simulink model "p4_car_colton_update1"  (R2025a)
settings: Solver=ode5  StartTime=0.0  StopTime=3600  FixedStep=0.001  RelTol=1e-3
undefined symbols (not defined in the file or in its folder): datBat, datCar, datMotor, path
libraries: slpidlib x1
settings Model: Creator=dxego  LastModifiedBy=umar
settings OptimizationCC: ReuseModelBlockBuffer=off
settings RTWCC: GPUComputeCapability=3.5

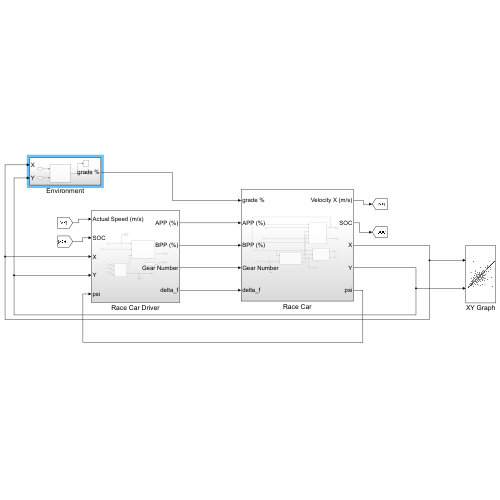
[thumbnail: Simulink's stored preview of the top-level diagram]
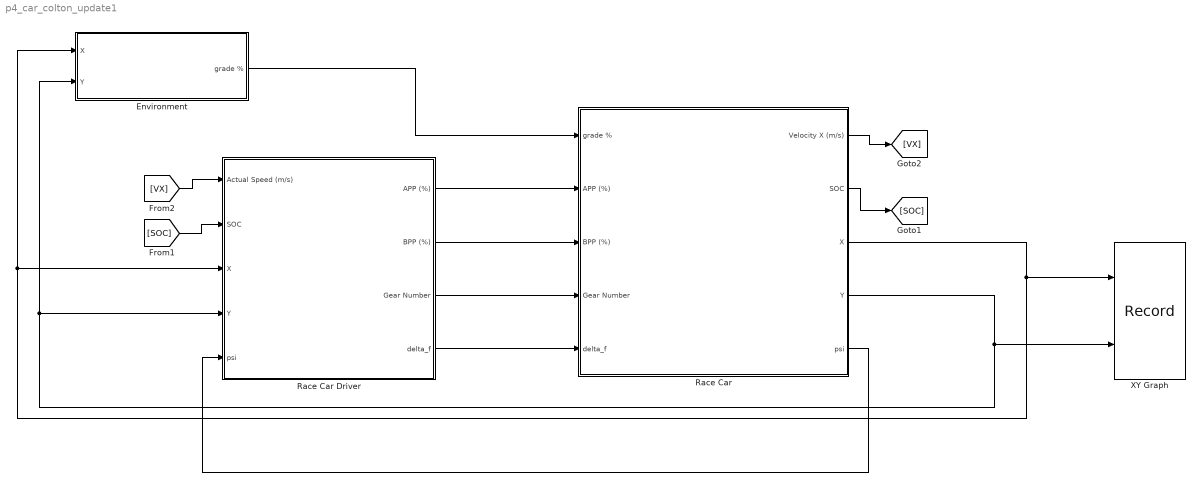
== system p4_car_colton_update1 ==
  Environment : Subsystem
  Race Car : Subsystem
  Race Car Driver : Subsystem
  XY Graph : Record  NumPorts=2.0  FileSettingsInternal="{\"entries\":[{\"content\":{\"excelSettings\":{\"content\":{},\"type\":\"Streamout.ExcelSettings\"},\"parquetSettings\":{\"content\":{},\"type\":\"Streamout.ParquetSettings\"}},\"type\":\"Streamout.FileSettingStorage\",\"uuid\":\"\"}],\"packageUris\":[\"http:\\/\\/schema.mathworks.com\\/mf0\\/streamout_blocks\\/R2020a\"],\"version\":\"1.0\"}"  FrameSettings=[0, 0]  Layout=[1 1]  SignalsInternal="{\"entries\":[{\"content\":{\"signals\":[{\"content\":{\"blockPath\":[],\"dimensions\":[1],\"domain\":\"\",\"lineColor\":\"#a2142f\",\"plots\":[ 1 ],\"port\":1,\"sid\":[\"\"],\"signalID\":1,\"signalName\":\"Race Car:3\"},\"type\":\"RecordBlkView.Signal\",\"uuid\":\"\"},{\"content\":{\"blockPath\":[],\"dimensions\":[1],\"domain\":\"\",\"lineColor\":\"#139fff\",\"plots\":[ 1 ],\"port\":2,\"sid\":[\"\"],\"signalID\":2,\"signalName\":\"Race Car:4\"},\"type\":\"RecordBlkView.Signal\",\"uuid\":\"\"}]},\"type\":\"RecordBlkView.InputSignals\",\"uuid\":\"\"}],\"packageUris\":[\"http:\\/\\/schema.mathworks.com\\/mf0\\/streamout_blocks\\/R2020a\"],\"version\":\"1.0\"}"  VisualizationBindings="{\"xyplotplugin\":{\"info\":[{\"series\":[{\"bindingParametersList\":[{\"parameter\":\"X-Axis\",\"signalID\":1,\"signalName\":\"Race Car:3\"},{\"parameter\":\"Y-Axis\",\"signalID\":2,\"signalName\":\"Race Car:4\"}],\"seriesID\":0}],\"subplotID\":1}]}}"  CompatibilityTag=XY  st=-1
  wires:
  [VX] -> Race Car Driver/1(Actual Speed (m/s))
  [SOC] -> Race Car Driver/2(SOC)
  Race Car/4(Y) -> XY Graph/2, Environment/2(Y), Race Car Driver/4(Y)
  Race Car/3(X) -> XY Graph/1, Environment/1(X), Race Car Driver/3(X)
  Race Car Driver/1(APP (%)) -> Race Car/2(APP (%))
  Race Car Driver/2(BPP (%)) -> Race Car/3("BPP (%) ")
  Race Car Driver/4(delta_f) -> Race Car/5(delta_f)
  Race Car/1(Velocity X (m/s)) -> [VX]
  Race Car/2(SOC) -> [SOC]
  Race Car Driver/3(Gear Number) -> Race Car/4(Gear Number)
  Environment/1(grade %) -> Race Car/1(grade %)
  Race Car/5(psi) -> Race Car Driver/5(psi)

== system p4_car_colton_update1/Environment ==
  X : Inport
  Y : Inport  Port=2
  MATLAB Function : MATLAB Function  TreatAsAtomicUnit=on
  Scope : Scope
      settings: ActiveDisplayYMinimum=-0.037768533551662917  ActiveDisplayYMaximum=0.038970623034102633  DataLoggingVariableName=ScopeData19
  grade % : Outport
  wires:
  X/1 -> MATLAB Function/1(x)
  Y/1 -> MATLAB Function/2(y)
  MATLAB Function/1(g) -> Scope/1, grade %/1

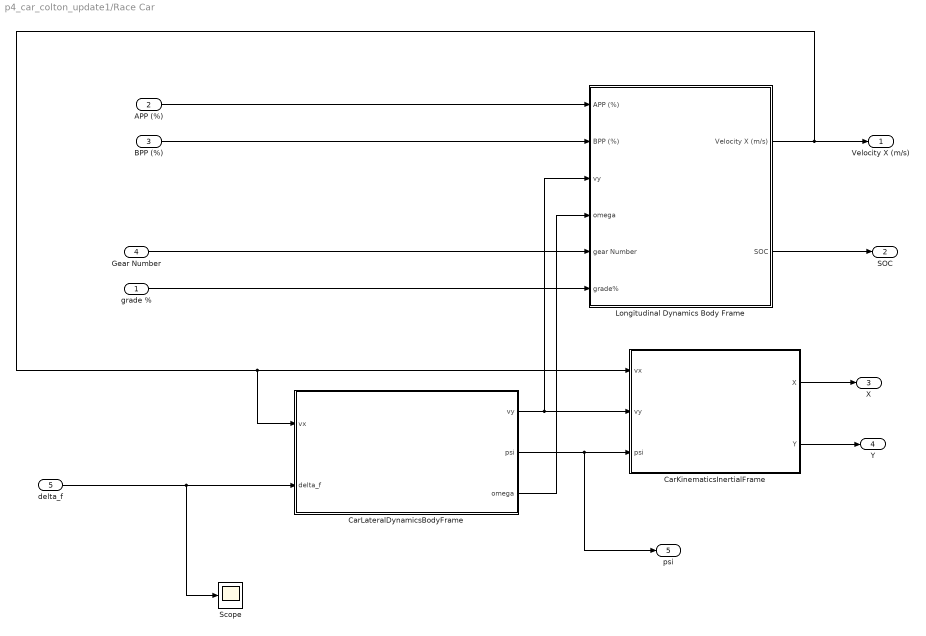
== system p4_car_colton_update1/Race Car ==
  grade % : Inport
  APP (%) : Inport  Port=2
  "BPP (%) " : Inport  Port=3
  Gear Number : Inport  Port=4
  delta_f : Inport  Port=5
  CarKinematicsInertialFrame : Subsystem
  CarLateralDynamicsBodyFrame : Subsystem
  Longitudinal Dynamics Body Frame : Subsystem
  Scope : Scope
      settings: ActiveDisplayYMinimum=-1.3496608820575011  ActiveDisplayYMaximum=9.010651011668978  DataLoggingVariableName=ScopeData16
  Velocity X (m/s) : Outport
  SOC : Outport  Port=2
  X : Outport  Port=3
  Y : Outport  Port=4
  psi : Outport  Port=5
  wires:
  CarKinematicsInertialFrame/2(Y) -> Y/1
  Longitudinal Dynamics Body Frame/2(SOC) -> SOC/1
  CarLateralDynamicsBodyFrame/2(psi) -> psi/1, CarKinematicsInertialFrame/3(psi)
  delta_f/1 -> Scope/1, CarLateralDynamicsBodyFrame/2(delta_f)
  APP (%)/1 -> Longitudinal Dynamics Body Frame/1(APP (%))
  CarLateralDynamicsBodyFrame/1(vy) -> Longitudinal Dynamics Body Frame/3(vy), CarKinematicsInertialFrame/2(vy)
  CarLateralDynamicsBodyFrame/3(omega) -> Longitudinal Dynamics Body Frame/4(omega)
  "BPP (%) "/1 -> Longitudinal Dynamics Body Frame/2("BPP (%) ")
  Longitudinal Dynamics Body Frame/1(Velocity X (m/s)) -> Velocity X (m/s)/1, CarLateralDynamicsBodyFrame/1(vx), CarKinematicsInertialFrame/1(vx)
  CarKinematicsInertialFrame/1(X) -> X/1
  Gear Number/1 -> Longitudinal Dynamics Body Frame/5(gear Number)
  grade %/1 -> Longitudinal Dynamics Body Frame/6(grade%)

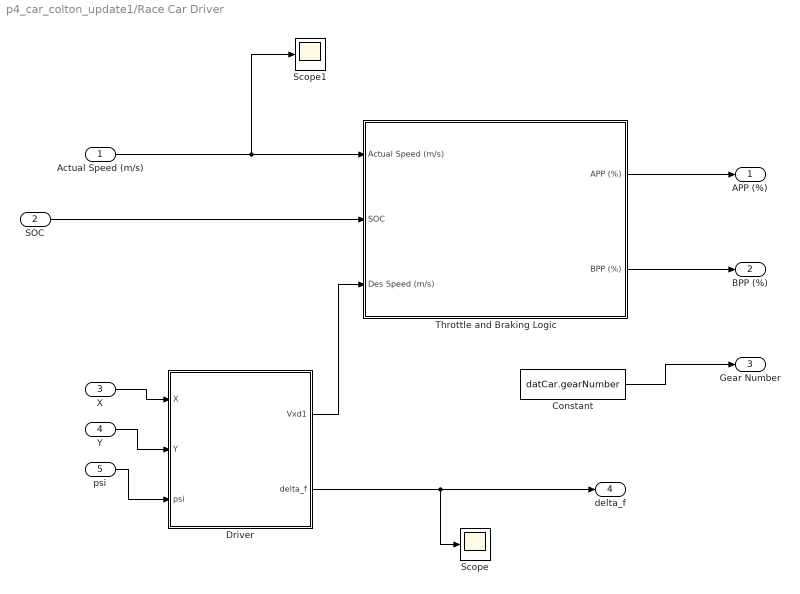
== system p4_car_colton_update1/Race Car Driver ==
  Actual Speed (m/s) : Inport
  SOC : Inport  Port=2
  X : Inport  Port=3
  Y : Inport  Port=4
  psi : Inport  Port=5
  Constant : Constant  Value=datCar.gearNumber
  Driver : Subsystem
  Scope : Scope
      settings: ActiveDisplayYMinimum=-1  ActiveDisplayYMaximum=1  DataLoggingVariableName=ScopeData12
  Scope1 : Scope
      settings: ActiveDisplayYMinimum=11.033893227651333  ActiveDisplayYMaximum=28.405080062704929  DataLoggingVariableName=ScopeData14
  "Throttle and Braking Logic " : Subsystem
  APP (%) : Outport
  BPP (%) : Outport  Port=2
  Gear Number : Outport  Port=3
  delta_f : Outport  Port=4
  wires:
  Y/1 -> Driver/2(Y)
  X/1 -> Driver/1(X)
  "Throttle and Braking Logic "/2(BPP (%)) -> BPP (%)/1
  Actual Speed (m/s)/1 -> Scope1/1, "Throttle and Braking Logic "/1(Actual Speed (m/s))
  "Throttle and Braking Logic "/1(APP (%)) -> APP (%)/1
  SOC/1 -> "Throttle and Braking Logic "/2(SOC)
  Driver/1(Vxd1) -> "Throttle and Braking Logic "/3("Des Speed (m/s) ")
  psi/1 -> Driver/3(psi)
  Constant/1 -> Gear Number/1
  Driver/2(delta_f) -> Scope/1, delta_f/1

== system p4_car_colton_update1/Race Car/CarKinematicsInertialFrame ==
  vx : Inport
  vy : Inport  Port=2
  psi : Inport  Port=3
  Integrator : Integrator  InitialCondition=datCar.init.X0
  Integrator1 : Integrator  InitialCondition=datCar.init.Y0
  KinematicVehicleModel_derivatives : MATLAB Function  TreatAsAtomicUnit=on  mask{obj=datCar}
      mask prompts: obj "obj structure"
  To Workspace : ToWorkspace  VariableName=X  SaveFormat=Timeseries  SampleTime=-1
  To Workspace1 : ToWorkspace  VariableName=Y  SaveFormat=Timeseries  SampleTime=-1
  X : Outport
  Y : Outport  Port=2
  wires:
  KinematicVehicleModel_derivatives/1(Xdot) -> Integrator/1
  KinematicVehicleModel_derivatives/2(Ydot) -> Integrator1/1
  Integrator/1 -> To Workspace/1, X/1
  Integrator1/1 -> Y/1, To Workspace1/1
  vx/1 -> KinematicVehicleModel_derivatives/1(vx)
  vy/1 -> KinematicVehicleModel_derivatives/2(vy)
  psi/1 -> KinematicVehicleModel_derivatives/3(psi)

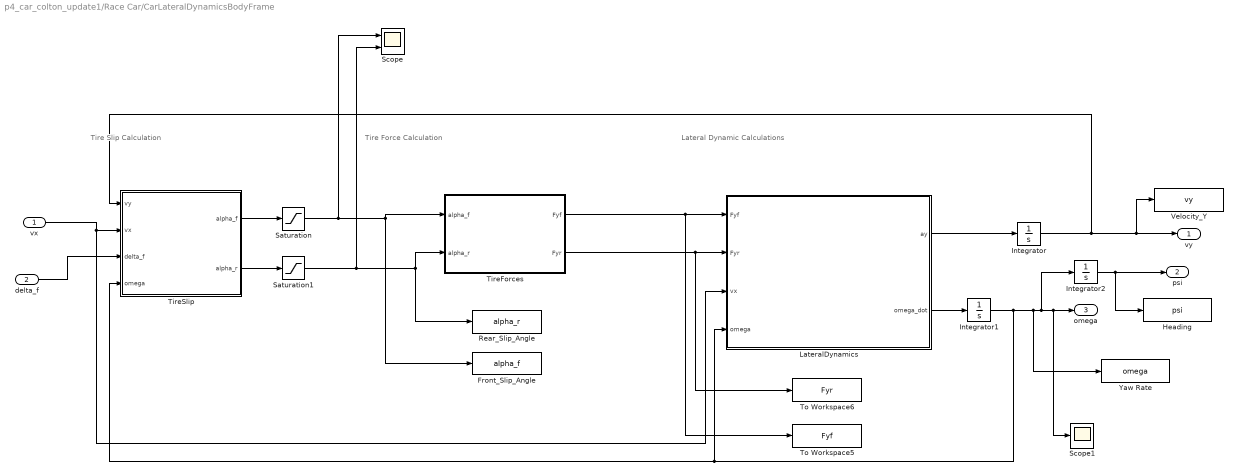
== system p4_car_colton_update1/Race Car/CarLateralDynamicsBodyFrame ==
  note: Tire Slip Calculation
  note: Tire Force Calculation
  note: Lateral Dynamic Calculations
  vx : Inport
  delta_f : Inport  Port=2
  Front_Slip_Angle : ToWorkspace  VariableName=alpha_f  SaveFormat=Timeseries  SampleTime=-1
  Heading : ToWorkspace  VariableName=psi  SaveFormat=Timeseries  SampleTime=-1
  Integrator : Integrator  InitialCondition=datCar.init.vy0
  Integrator1 : Integrator  InitialCondition=datCar.init.omega0
  Integrator2 : Integrator  InitialCondition=datCar.init.psi0
  LateralDynamics : MATLAB Function  TreatAsAtomicUnit=on  mask{obj=datCar}
      mask prompts: obj "obj structure"
  Rear_Slip_Angle : ToWorkspace  VariableName=alpha_r  SaveFormat=Timeseries  SampleTime=-1
  Saturation : Saturate  UpperLimit=datCar.maxAlpha  LowerLimit=-datCar.maxAlpha
  Saturation1 : Saturate  UpperLimit=datCar.maxAlpha  LowerLimit=-datCar.maxAlpha
  Scope : Scope  NumInputPorts=2
      settings: ActiveDisplayYMinimum=-1  ActiveDisplayYMaximum=1  DataLoggingVariableName=ScopeData13
  Scope1 : Scope
      settings: ActiveDisplayYMinimum=-1  ActiveDisplayYMaximum=1  DataLoggingVariableName=ScopeData17
  TireForces : MATLAB Function  TreatAsAtomicUnit=on  mask{obj=datCar}
      mask prompts: obj "obj structure"
  TireSlip : MATLAB Function  TreatAsAtomicUnit=on  mask{obj=datCar}
      mask prompts: obj "obj structure"
  To Workspace5 : ToWorkspace  VariableName=Fyf  SaveFormat=Timeseries  SampleTime=-1
  To Workspace6 : ToWorkspace  VariableName=Fyr  SaveFormat=Timeseries  SampleTime=-1
  Velocity_Y : ToWorkspace  VariableName=vy  SaveFormat=Timeseries  SampleTime=-1
  Yaw Rate : ToWorkspace  VariableName=omega  SaveFormat=Timeseries  SampleTime=-1
  vy : Outport
  psi : Outport  Port=2
  omega : Outport  Port=3
  wires:
  LateralDynamics/1(ay) -> Integrator/1
  Integrator/1 -> vy/1, Velocity_Y/1, TireSlip/1(vy)
  LateralDynamics/2(omega_dot) -> Integrator1/1
  Integrator1/1 -> Integrator2/1, Scope1/1, omega/1, Yaw Rate/1, LateralDynamics/4(omega), TireSlip/4(omega)
  TireSlip/1(alpha_f) -> Saturation/1
  TireSlip/2(alpha_r) -> Saturation1/1
  TireForces/1(Fyf) -> LateralDynamics/1(Fyf), To Workspace5/1
  TireForces/2(Fyr) -> LateralDynamics/2(Fyr), To Workspace6/1
  Saturation/1 -> Scope/1, TireForces/1(alpha_f), Front_Slip_Angle/1
  Saturation1/1 -> Scope/2, TireForces/2(alpha_r), Rear_Slip_Angle/1
  vx/1 -> TireSlip/2(vx), LateralDynamics/3(vx)
  delta_f/1 -> TireSlip/3(delta_f)
  Integrator2/1 -> Heading/1, psi/1

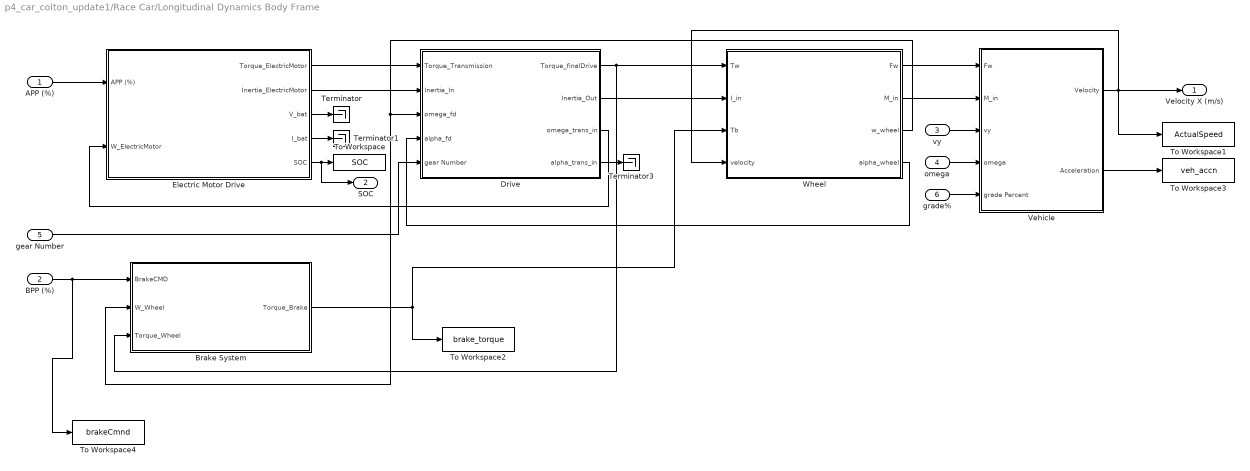
== system p4_car_colton_update1/Race Car/Longitudinal Dynamics Body Frame ==
  APP (%) : Inport
  "BPP (%) " : Inport  Port=2
  vy : Inport  Port=3
  omega : Inport  Port=4
  gear Number : Inport  Port=5
  grade% : Inport  Port=6
  Brake System : Subsystem
  Drive : Subsystem
  Electric Motor Drive : Subsystem
  Terminator : Terminator
  Terminator1 : Terminator
  Terminator3 : Terminator
  To Workspace : ToWorkspace  VariableName=SOC  SaveFormat=Timeseries  SampleTime=-1
  To Workspace1 : ToWorkspace  VariableName=ActualSpeed  SaveFormat=Timeseries  SampleTime=-1
  To Workspace2 : ToWorkspace  VariableName=brake_torque  SaveFormat=Timeseries  SampleTime=-1
  To Workspace3 : ToWorkspace  VariableName=veh_accn  SaveFormat=Timeseries  SampleTime=-1
  To Workspace4 : ToWorkspace  VariableName=brakeCmnd  SaveFormat=Timeseries  SampleTime=-1
  Vehicle : Subsystem
  "Wheel " : Subsystem
  Velocity X (m/s) : Outport
  SOC : Outport  Port=2
  wires:
  Drive/3(omega_trans_in) -> Electric Motor Drive/2(W_ElectricMotor)
  Electric Motor Drive/2(Inertia_ElectricMotor) -> Drive/2(Inertia_In)
  Electric Motor Drive/3(V_bat) -> Terminator/1
  Vehicle/2(Acceleration) -> To Workspace3/1
  Drive/1(Torque_finalDrive) -> "Wheel "/1(Tw), Brake System/3(Torque_Wheel)
  Electric Motor Drive/1(Torque_ElectricMotor) -> Drive/1(Torque_Transmission)
  Drive/2(Inertia_Out) -> "Wheel "/2(I_in)
  "Wheel "/2(M_in) -> Vehicle/2("M_in ")
  "BPP (%) "/1 -> To Workspace4/1, Brake System/1("BrakeCMD ")
  "Wheel "/3(w_wheel) -> Brake System/2(W_Wheel), Drive/3(omega_fd)
  "Wheel "/1(Fw) -> Vehicle/1(Fw)
  Brake System/1(Torque_Brake) -> To Workspace2/1, "Wheel "/3(Tb)
  Drive/4(alpha_trans_in) -> Terminator3/1
  "Wheel "/4(alpha_wheel) -> Drive/4(alpha_fd)
  Electric Motor Drive/4(I_bat) -> Terminator1/1
  APP (%)/1 -> Electric Motor Drive/1(APP (%))
  vy/1 -> Vehicle/3(vy)
  omega/1 -> Vehicle/4(omega)
  Vehicle/1("Velocity ") -> "Wheel "/4(velocity), Velocity X (m/s)/1, To Workspace1/1
  Electric Motor Drive/5(SOC) -> SOC/1, To Workspace/1
  gear Number/1 -> Drive/5(gear Number)
  grade%/1 -> Vehicle/5(grade Percent)

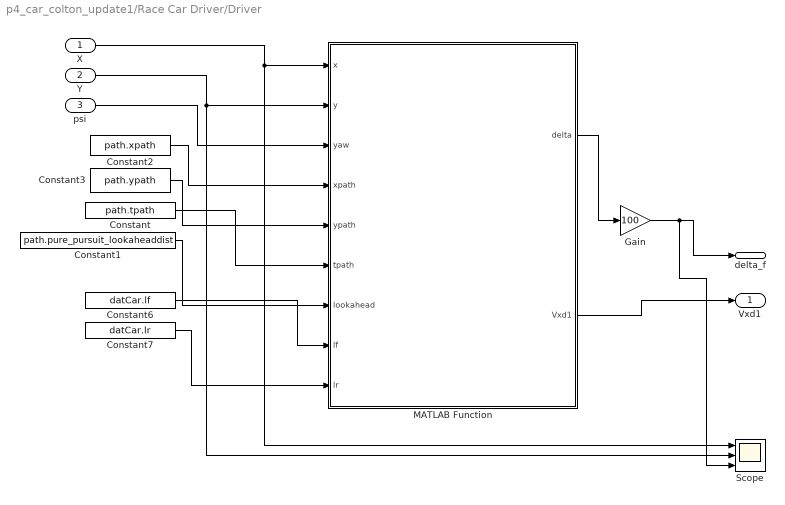
== system p4_car_colton_update1/Race Car Driver/Driver ==
  X : Inport
  Y : Inport  Port=2
  psi : Inport  Port=3
  Constant : Constant  Value=path.tpath
  Constant1 : Constant  Value=path.pure_pursuit_lookaheaddist
  Constant2 : Constant  Value=path.xpath
  Constant3 : Constant  Value=path.ypath
  Constant6 : Constant  Value=datCar.lf
  Constant7 : Constant  Value=datCar.lr
  Gain : Gain  Gain=100
  MATLAB Function : MATLAB Function  TreatAsAtomicUnit=on
  Scope : Scope  NumInputPorts=3
      settings: ActiveDisplayYMinimum=-137.49213624230239  ActiveDisplayYMaximum=1237.4292261807218
  Vxd1 : Outport
  delta_f : Outport  Port=2
  wires:
  X/1 -> Scope/1, MATLAB Function/1(x)
  Y/1 -> Scope/2, MATLAB Function/2(y)
  psi/1 -> MATLAB Function/3(yaw)
  MATLAB Function/2(Vxd1) -> Vxd1/1
  Constant2/1 -> MATLAB Function/4(xpath)
  Constant3/1 -> MATLAB Function/5(ypath)
  Constant/1 -> MATLAB Function/6(tpath)
  Constant1/1 -> MATLAB Function/7(lookahead)
  Constant6/1 -> MATLAB Function/8(lf)
  Constant7/1 -> MATLAB Function/9(lr)
  MATLAB Function/1(delta) -> Gain/1
  Gain/1 -> Scope/3, delta_f/1

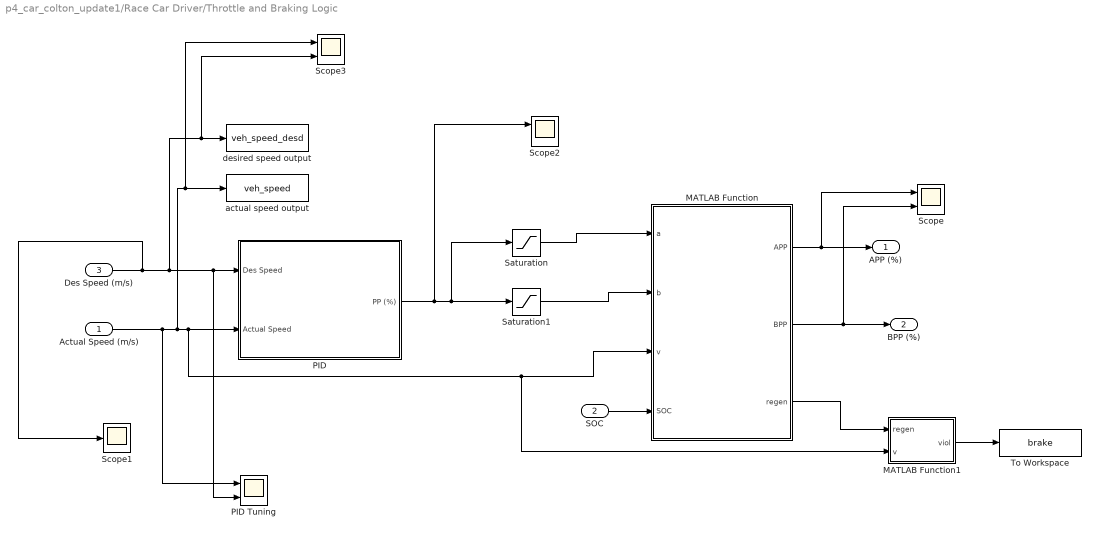
== system p4_car_colton_update1/Race Car Driver/Throttle and Braking Logic  ==
  Actual Speed (m/s) : Inport
  SOC : Inport  Port=2
  "Des Speed (m/s) " : Inport  Port=3
  MATLAB Function : MATLAB Function  TreatAsAtomicUnit=on
  MATLAB Function1 : MATLAB Function  TreatAsAtomicUnit=on
  PID : Subsystem
  PID Tuning : Scope  NumInputPorts=2
      settings: ActiveDisplayYMinimum=-4.40832  ActiveDisplayYMaximum=37.63006
  Saturation : Saturate  UpperLimit=1  LowerLimit=0
  Saturation1 : Saturate  UpperLimit=0  LowerLimit=-1
  Scope : Scope  NumInputPorts=2
      settings: ActiveDisplayYMinimum=-1.0607  ActiveDisplayYMaximum=1.06103
  Scope1 : Scope
      settings: ActiveDisplayYMinimum=-1  ActiveDisplayYMaximum=1  DataLoggingVariableName=ScopeData15
  Scope2 : Scope  NumInputPorts=2
      settings: ActiveDisplayYMinimum=-1.0607  ActiveDisplayYMaximum=1.06103  DataLoggingVariableName=ScopeData5
  Scope3 : Scope  NumInputPorts=2
      settings: ActiveDisplayYMinimum=27.321282013339456  ActiveDisplayYMaximum=39.0725745132226  DataLoggingVariableName=ScopeData11
  To Workspace : ToWorkspace  VariableName=brake  SaveFormat=Timeseries  SampleTime=-1
  actual speed output : ToWorkspace  VariableName=veh_speed  SaveFormat=Timeseries  SampleTime=-1
  desired speed output : ToWorkspace  VariableName=veh_speed_desd  SaveFormat=Timeseries  SampleTime=-1
  APP (%) : Outport
  BPP (%) : Outport  Port=2
  wires:
  PID/1(PP (%)) -> Scope2/1, Saturation1/1, Saturation/1
  Saturation1/1 -> MATLAB Function/2(b)
  Actual Speed (m/s)/1 -> PID Tuning/1, actual speed output/1, Scope3/1, MATLAB Function1/2(v), MATLAB Function/3(v), PID/2(Actual Speed)
  "Des Speed (m/s) "/1 -> Scope1/1, PID Tuning/2, PID/1("Des Speed "), Scope3/2, desired speed output/1
  Saturation/1 -> MATLAB Function/1(a)
  MATLAB Function/1(APP) -> Scope/1, APP (%)/1
  MATLAB Function/2(BPP) -> Scope/2, BPP (%)/1
  MATLAB Function1/1(viol) -> To Workspace/1
  SOC/1 -> MATLAB Function/4(SOC)
  MATLAB Function/3(regen) -> MATLAB Function1/1(regen)

== system p4_car_colton_update1/Race Car/Longitudinal Dynamics Body Frame/Brake System ==
  "BrakeCMD " : Inport
  W_Wheel : Inport  Port=2
  Torque_Wheel : Inport  Port=3
  Brake Torque : MATLAB Function  TreatAsAtomicUnit=on
  Constant : Constant  Value=datCar.maxBrakeTorque
  Scope : Scope
      settings: ActiveDisplayYMinimum=-3252.17168  ActiveDisplayYMaximum=56.62718  DataLoggingVariableName=ScopeData4
  Torque_Brake : Outport  VectorParamsAs1DForOutWhenUnconnected=off
  wires:
  "BrakeCMD "/1 -> Brake Torque/1(BBcmd)
  Brake Torque/1(Tb) -> Scope/1, Torque_Brake/1
  W_Wheel/1 -> Brake Torque/3(w_wheel)
  Constant/1 -> Brake Torque/2(Tbcap)

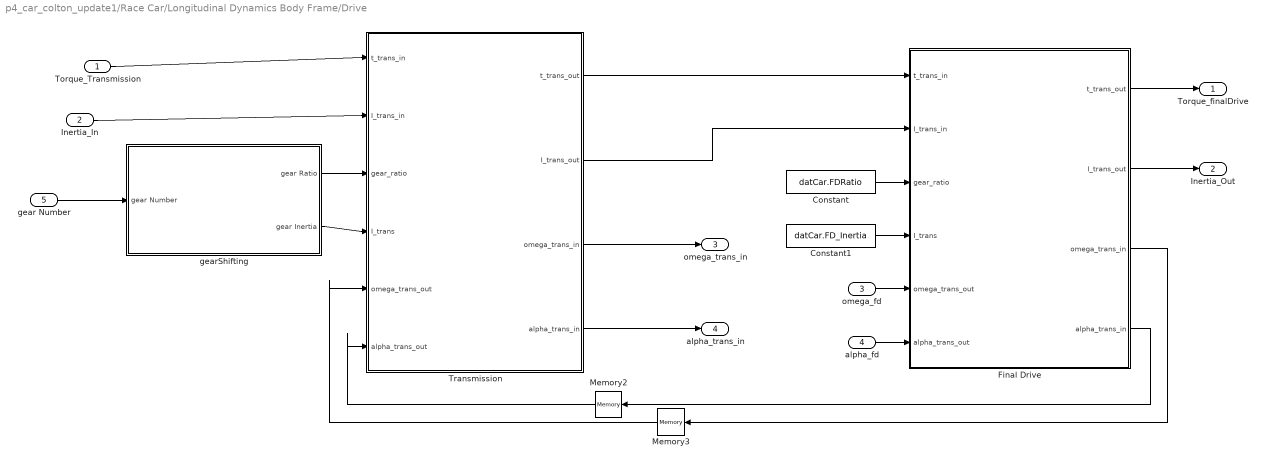
== system p4_car_colton_update1/Race Car/Longitudinal Dynamics Body Frame/Drive ==
  Torque_Transmission : Inport
  Inertia_In : Inport  Port=2
  omega_fd : Inport  Port=3
  alpha_fd : Inport  Port=4
  gear Number : Inport  Port=5
  Constant : Constant  Value=datCar.FDRatio
  Constant1 : Constant  Value=datCar.FD_Inertia
  Final Drive : MATLAB Function  TreatAsAtomicUnit=on
  Memory2 : Memory
  Memory3 : Memory
  Transmission : MATLAB Function  TreatAsAtomicUnit=on
  gearShifting : Subsystem
  Torque_finalDrive : Outport
  Inertia_Out : Outport  Port=2
  omega_trans_in : Outport  Port=3
  alpha_trans_in : Outport  Port=4
  wires:
  Final Drive/4(alpha_trans_in) -> Memory2/1
  Final Drive/3(omega_trans_in) -> Memory3/1
  Transmission/1(t_trans_out) -> Final Drive/1(t_trans_in)
  Transmission/2(I_trans_out) -> Final Drive/2(I_trans_in)
  Transmission/4(alpha_trans_in) -> alpha_trans_in/1
  Final Drive/1(t_trans_out) -> Torque_finalDrive/1
  Final Drive/2(I_trans_out) -> Inertia_Out/1
  omega_fd/1 -> Final Drive/5(omega_trans_out)
  alpha_fd/1 -> Final Drive/6(alpha_trans_out)
  Constant/1 -> Final Drive/3(gear_ratio)
  Constant1/1 -> Final Drive/4(I_trans)
  gear Number/1 -> gearShifting/1(gear Number)
  gearShifting/1(gear Ratio) -> Transmission/3(gear_ratio)
  gearShifting/2(gear Inertia) -> Transmission/4(I_trans)
  Inertia_In/1 -> Transmission/2(I_trans_in)
  Transmission/3(omega_trans_in) -> omega_trans_in/1
  Torque_Transmission/1 -> Transmission/1(t_trans_in)
  Memory2/1 -> Transmission/6(alpha_trans_out)
  Memory3/1 -> Transmission/5(omega_trans_out)

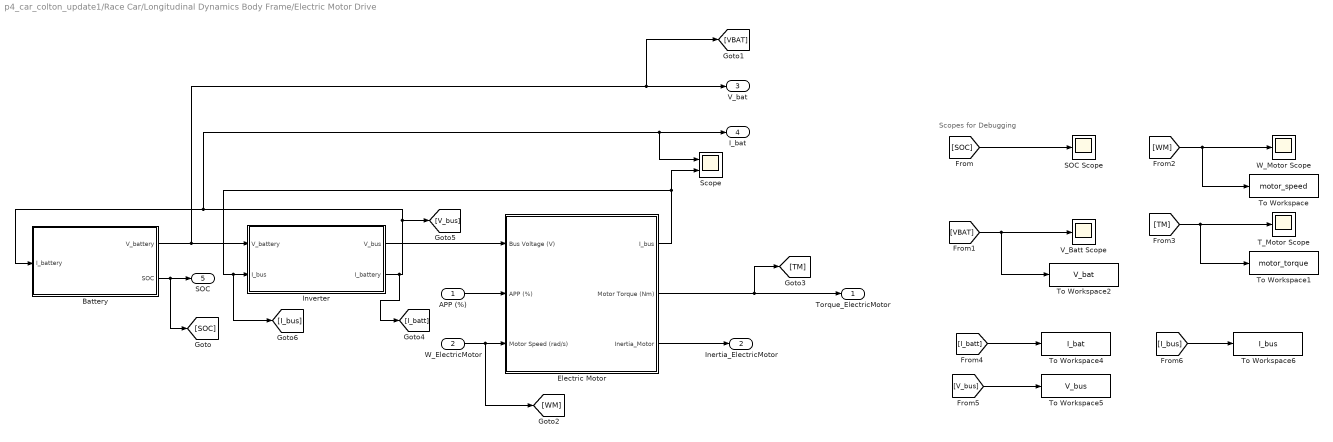
== system p4_car_colton_update1/Race Car/Longitudinal Dynamics Body Frame/Electric Motor Drive ==
  note: Scopes for Debugging
  APP (%) : Inport
  W_ElectricMotor : Inport  Port=2
  Battery : Subsystem
  Electric Motor : Subsystem
  Inverter : Subsystem
  SOC Scope : Scope
      settings: ActiveDisplayYMinimum=0.79068  ActiveDisplayYMaximum=0.80103  DataLoggingVariableName=ScopeData7
  Scope : Scope  NumInputPorts=2
      settings: ActiveDisplayYMinimum=-92.41521  ActiveDisplayYMaximum=118.26537  DataLoggingVariableName=ScopeData2
  T_Motor Scope : Scope
      settings: ActiveDisplayYMinimum=-92.74121  ActiveDisplayYMaximum=115.47111  DataLoggingVariableName=ScopeData10
  To Workspace : ToWorkspace  VariableName=motor_speed  SaveFormat=Timeseries  SampleTime=-1
  To Workspace1 : ToWorkspace  VariableName=motor_torque  SaveFormat=Timeseries  SampleTime=-1
  To Workspace2 : ToWorkspace  VariableName=V_bat  SaveFormat=Timeseries  SampleTime=-1
  To Workspace4 : ToWorkspace  VariableName=I_bat  SaveFormat=Timeseries  SampleTime=-1
  To Workspace5 : ToWorkspace  VariableName=V_bus  SaveFormat=Timeseries  SampleTime=-1
  To Workspace6 : ToWorkspace  VariableName=I_bus  SaveFormat=Timeseries  SampleTime=-1
  V_Batt Scope : Scope
      settings: ActiveDisplayYMinimum=354.15627  ActiveDisplayYMaximum=391.49042  DataLoggingVariableName=ScopeData8
  W_Motor Scope : Scope
      settings: ActiveDisplayYMinimum=-83.74997  ActiveDisplayYMaximum=695.87961  DataLoggingVariableName=ScopeData9
  Torque_ElectricMotor : Outport
  Inertia_ElectricMotor : Outport  Port=2
  V_bat : Outport  Port=3
  I_bat : Outport  Port=4
  SOC : Outport  Port=5
  wires:
  APP (%)/1 -> Electric Motor/2(APP (%))
  W_ElectricMotor/1 -> [WM], Electric Motor/3(Motor Speed (rad/s))
  Electric Motor/3(Inertia_Motor) -> Inertia_ElectricMotor/1
  Inverter/1(V_bus) -> Electric Motor/1(Bus Voltage (V))
  Inverter/2(I_battery) -> [I_batt], Scope/1, I_bat/1, Battery/1(I_battery), [V_bus]
  Electric Motor/1(I_bus) -> Scope/2, [I_bus], Inverter/2(I_bus)
  [SOC] -> SOC Scope/1
  [VBAT] -> To Workspace2/1, V_Batt Scope/1
  [WM] -> To Workspace/1, W_Motor Scope/1
  [TM] -> To Workspace1/1, T_Motor Scope/1
  Battery/1(V_battery) -> [VBAT], V_bat/1, Inverter/1(V_battery)
  Electric Motor/2(Motor Torque (Nm)) -> [TM], Torque_ElectricMotor/1
  Battery/2(SOC) -> [SOC], SOC/1
  [I_batt] -> To Workspace4/1
  [V_bus] -> To Workspace5/1
  [I_bus] -> To Workspace6/1

== system p4_car_colton_update1/Race Car/Longitudinal Dynamics Body Frame/Vehicle ==
  Fw : Inport
  "M_in " : Inport  Port=2
  vy : Inport  Port=3
  omega : Inport  Port=4
  grade Percent : Inport  Port=5
  vehicleDragForce : Subsystem
  vehicleDynamics : Subsystem
  "Velocity " : Outport  VectorParamsAs1DForOutWhenUnconnected=off
  Acceleration : Outport  Port=2
  wires:
  vehicleDynamics/2(Out2) -> vehicleDragForce/1(vel), "Velocity "/1
  Fw/1 -> vehicleDynamics/1("Fw ")
  vehicleDragForce/1(Fdrag) -> vehicleDynamics/2(Fd)
  "M_in "/1 -> vehicleDynamics/3("M_in ")
  vy/1 -> vehicleDynamics/4(vy)
  omega/1 -> vehicleDynamics/5(omega)
  vehicleDynamics/1(acceleration) -> Acceleration/1
  grade Percent/1 -> vehicleDynamics/6(grade Percent)

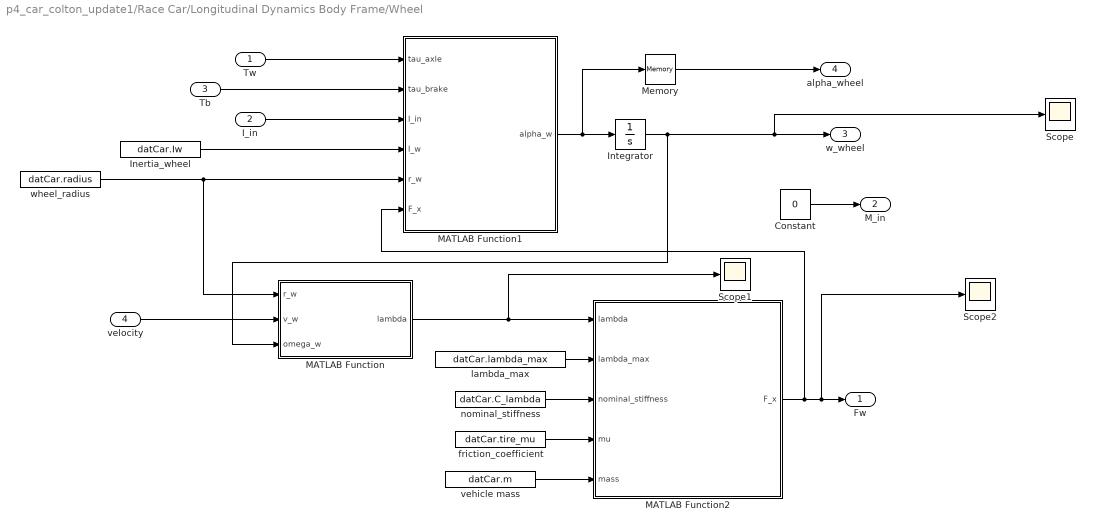
== system p4_car_colton_update1/Race Car/Longitudinal Dynamics Body Frame/Wheel  ==
  Tw : Inport
  I_in : Inport  Port=2
  Tb : Inport  Port=3
  velocity : Inport  Port=4
  Constant : Constant  Value=0
  Inertia_wheel : Constant  Value=datCar.Iw
  Integrator : Integrator  InitialCondition=datCar.init.omega0
  MATLAB Function : MATLAB Function  TreatAsAtomicUnit=on
  MATLAB Function1 : MATLAB Function  TreatAsAtomicUnit=on
  MATLAB Function2 : MATLAB Function  TreatAsAtomicUnit=on
  Memory : Memory
  Scope : Scope
      settings: ActiveDisplayYMinimum=-11.16666  ActiveDisplayYMaximum=92.78395
  Scope1 : Scope
      settings: ActiveDisplayYMinimum=-33.74112  ActiveDisplayYMaximum=2.76989  DataLoggingVariableName=ScopeData2
  Scope2 : Scope
      settings: ActiveDisplayYMinimum=-88.22724  ActiveDisplayYMaximum=2.56826  DataLoggingVariableName=ScopeData3
  friction_coefficient : Constant  Value=datCar.tire_mu
  lambda_max : Constant  Value=datCar.lambda_max
  nominal_stiffness : Constant  Value=datCar.C_lambda
  vehicle mass : Constant  Value=datCar.m
  wheel_radius : Constant  Value=datCar.radius
  Fw : Outport
  M_in : Outport  Port=2
  w_wheel : Outport  Port=3
  alpha_wheel : Outport  Port=4
  wires:
  velocity/1 -> MATLAB Function/2(v_w)
  Tw/1 -> MATLAB Function1/1(tau_axle)
  Tb/1 -> MATLAB Function1/2(tau_brake)
  I_in/1 -> MATLAB Function1/3(I_in)
  Inertia_wheel/1 -> MATLAB Function1/4(I_w)
  wheel_radius/1 -> MATLAB Function/1(r_w), MATLAB Function1/5(r_w)
  MATLAB Function1/1(alpha_w) -> Memory/1, Integrator/1
  Integrator/1 -> MATLAB Function/3(omega_w), Scope/1, w_wheel/1
  MATLAB Function/1(lambda) -> Scope1/1, MATLAB Function2/1(lambda)
  nominal_stiffness/1 -> MATLAB Function2/3(nominal_stiffness)
  lambda_max/1 -> MATLAB Function2/2(lambda_max)
  friction_coefficient/1 -> MATLAB Function2/4(mu)
  vehicle mass/1 -> MATLAB Function2/5(mass)
  MATLAB Function2/1(F_x) -> Scope2/1, Fw/1, MATLAB Function1/6(F_x)
  Constant/1 -> M_in/1
  Memory/1 -> alpha_wheel/1

== system p4_car_colton_update1/Race Car Driver/Throttle and Braking Logic /PID ==
  "Des Speed " : Inport
  Actual Speed : Inport  Port=2
  PID Controller : slpidlib/PID Controller  Controller=PID  Form=Parallel  TimeDomain=Continuous-time  UseExternalTs=off  SampleTime=-1  IntegratorMethod=Forward Euler  FilterMethod=Forward Euler  ControllerParametersSource=internal  P=0.4  I=0.05  UseKiTs=off  D=0.01  UseExternalDerivativeSource=off  N=100  UseFilter=on  TunerSelectOption=Transfer Function Based (PID Tuner App)  InitialConditionSource=internal  InitialConditionForIntegrator=0  InitialConditionForFilter=0  DifferentiatorICPrevScaledInput=0  ExternalReset=none  TrackingMode=off  Kt=1  LimitOutput=off  SatLimitsSource=internal  UpperSaturationLimit=inf  LowerSaturationLimit=-inf  LinearizeAsGain=on  AntiWindupMode=none  Kb=1  LimitIntegrator=off  UpperIntegratorSaturationLimit=inf  LowerIntegratorSaturationLimit=-inf  POutMin=[]  POutMax=[]  IOutMin=[]  IOutMax=[]  DOutMin=[]  DOutMax=[]  NOutMin=[]  NOutMax=[]  SumOutMin=[]  SumOutMax=[]  SaturationOutMin=[]  SaturationOutMax=[]  PParamMin=[]  PParamMax=[]  IParamMin=[]  IParamMax=[]  DParamMin=[]  DParamMax=[]  NParamMin=[]  NParamMax=[]  KbParamMin=[]  KbParamMax=[]  KtParamMin=[]  KtParamMax=[]  KbOutMin=[]  KbOutMax=[]  KtOutMin=[]  KtOutMax=[]  IntegratorOutMin=[]  IntegratorOutMax=[]  FilterOutMin=[]  FilterOutMax=[]  SumI1OutMin=[]  SumI1OutMax=[]  SumI2OutMin=[]  SumI2OutMax=[]  SumI3OutMin=[]  SumI3OutMax=[]  SumI4OutMin=[]  SumI4OutMax=[]  SumDOutMin=[]  SumDOutMax=[]  DifferentiatorOutMin=[]  DifferentiatorOutMax=[]  FilterDiffOutCoefMin=[]  FilterDiffOutCoefMax=[]  ReciprocalOutMin=[]  ReciprocalOutMax=[]  SumDenOutMin=[]  SumDenOutMax=[]  SumNumOutMin=[]  SumNumOutMax=[]  DivideOutMin=[]  DivideOutMax=[]  UdiffTsProdOutMin=[]  UdiffTsProdOutMax=[]  NTsProdOutMin=[]  NTsProdOutMax=[]  UintegralTsProdOutMin=[]  UintegralTsProdOutMax=[]  UngainTsProdOutMin=[]  UngainTsProdOutMax=[]  ClampingZeroOutDataTypeStr=Inherit: Inherit via back propagation  ClampingZeroOutMin=[]  ClampingZeroOutMax=[]  FilterDenConstantOutDataTypeStr=Inherit: Inherit via back propagation  FilterDenConstantOutMin=[]  FilterDenConstantOutMax=[]  PCopyOutDataTypeStr=Inherit: Inherit via back propagation  PCopyOutMin=[]  PCopyOutMax=[]  NCopyOutDataTypeStr=Inherit: Inherit via back propagation  NCopyOutMin=[]  NCopyOutMax=[]  IntegratorContinuousStateAttributes=''  IntegratorStateMustResolveToSignalObject=off  IntegratorRTWStateStorageClass=Auto  FilterContinuousStateAttributes=''  FilterStateMustResolveToSignalObject=off  FilterRTWStateStorageClass=Auto  ParallelPVariant=InternalParameters  IdealPVariant=Disabled  IVariant=InternalParameters  DVariant=InternalParameters  IntegratorVariant=Continuous  SatVariant=Disabled  AWVariant=Passthrough  PCopyVariant=Disabled  TRVariant=Disabled  FdbkBlocksVariant=Forward  IdealPFdbkVariant=Disabled  SatFdbkVariant=Disabled  DerivativeFilterVariant=ContFilter  NVariant=InternalParameters  NCopyVariant=Disabled  FilterICVariant=InternalICsFilter  IntegratorICVariant=InternalICs  ExternalResetVariant=Disabled  TRSumVariant=Passthrough  SumFdbkVariant=Disabled  SumVariant=Sum_PID  TsampFilterVariant=InternalTs  TsampNgainVariant=Passthrough  TsampIntegralVariant=Disabled_SignalSpec  ExternalSaturationOutDataTypeStr=Inherit: Same as second input  DerivativeSourceVariant=ErrorSignal  PreIntVariant=InternalPreInt
  Sum : Sum  Inputs=|+-
  To Workspace : ToWorkspace  VariableName=v_error  SaveFormat=Timeseries  SampleTime=-1
  PP (%) : Outport
  wires:
  Sum/1 -> PID Controller/1, To Workspace/1
  "Des Speed "/1 -> Sum/1
  Actual Speed/1 -> Sum/2
  PID Controller/1 -> PP (%)/1

== system p4_car_colton_update1/Race Car/Longitudinal Dynamics Body Frame/Drive/gearShifting ==
  gear Number : Inport
  Rate Limiter : RateLimiter  SampleTimeMode=inherited
  Rate Limiter1 : RateLimiter  SampleTimeMode=inherited
  gear Inertia calc : Lookup_n-D  NumberOfTableDimensions=1  BreakpointsForDimension1=datCar.gear.gearNumbers  Table=datCar.gear.gearInertias  InternalRulePriority=Speed  RndMeth=Simplest
  gear Ratio calc : Lookup_n-D  NumberOfTableDimensions=1  BreakpointsForDimension1=datCar.gear.gearNumbers  Table=datCar.gear.gearRatios  InternalRulePriority=Speed  RndMeth=Simplest
  gear Ratio : Outport
  gear Inertia : Outport  Port=2
  wires:
  gear Inertia calc/1 -> Rate Limiter1/1
  gear Number/1 -> gear Inertia calc/1, gear Ratio calc/1
  gear Ratio calc/1 -> Rate Limiter/1
  Rate Limiter1/1 -> gear Inertia/1
  Rate Limiter/1 -> gear Ratio/1

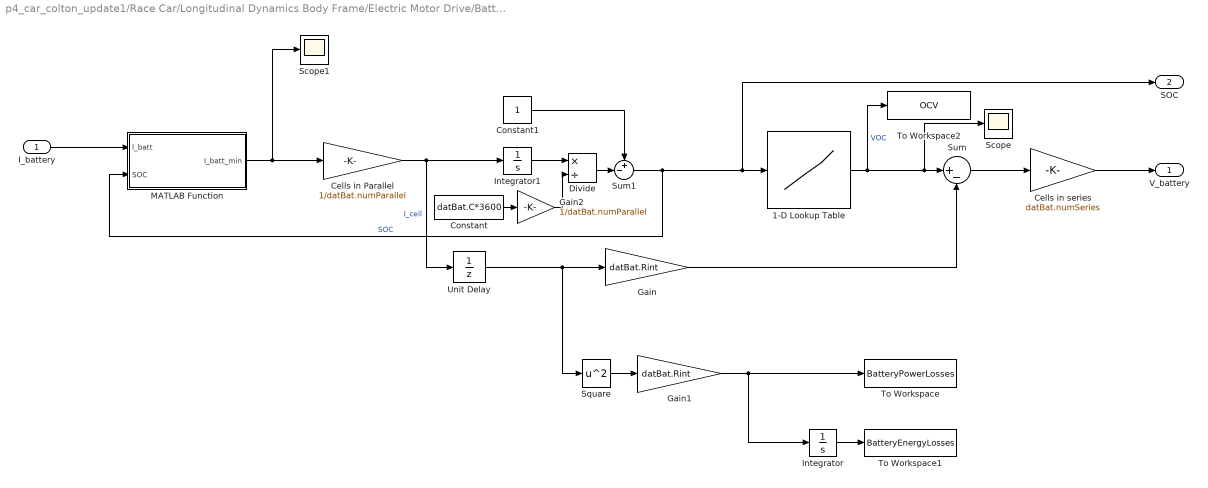
== system p4_car_colton_update1/Race Car/Longitudinal Dynamics Body Frame/Electric Motor Drive/Battery ==
  I_battery : Inport
  1-D Lookup Table : Lookup_n-D  NumberOfTableDimensions=1  BreakpointsForDimension1=datBat.SOC  Table=datBat.OCV  ExtrapMethod=Clip  UseLastTableValue=on  InternalRulePriority=Speed  RndMeth=Simplest
  Cells in Parallel : Gain  Gain=1/datBat.numParallel
  Cells in series : Gain  Gain=datBat.numSeries
  Constant : Constant  Value=datBat.C*3600
  Constant1 : Constant
  Divide : Product  Inputs=*/
  Gain : Gain  Gain=datBat.Rint
  Gain1 : Gain  Gain=datBat.Rint
  Gain2 : Gain  Gain=1/datBat.numParallel
  Integrator : Integrator
  Integrator1 : Integrator  InitialCondition=1459.5
  MATLAB Function : MATLAB Function  TreatAsAtomicUnit=on
  Scope : Scope
      settings: ActiveDisplayYMinimum=3.94534  ActiveDisplayYMaximum=3.95051  DataLoggingVariableName=ScopeData5
  Scope1 : Scope
      settings: ActiveDisplayYMinimum=-13642.01405  ActiveDisplayYMaximum=120182.56485  DataLoggingVariableName=ScopeData6
  Square : Math  Operator=square
  Sum : Sum  Inputs=|+-
  Sum1 : Sum  Inputs=+-|
  To Workspace : ToWorkspace  VariableName=BatteryPowerLosses  SaveFormat=Timeseries  SampleTime=-1
  To Workspace1 : ToWorkspace  VariableName=BatteryEnergyLosses  SaveFormat=Timeseries  SampleTime=-1
  To Workspace2 : ToWorkspace  VariableName=OCV  SaveFormat=Timeseries  SampleTime=-1
  Unit Delay : UnitDelay  SampleTime=-1  HasFrameUpgradeWarning=on
  V_battery : Outport
  SOC : Outport  Port=2
  wires:
  Cells in Parallel/1 -> Integrator1/1, Unit Delay/1  "I_cell"
  Sum1/1 -> MATLAB Function/2(SOC), SOC/1, 1-D Lookup Table/1  "SOC"
  1-D Lookup Table/1 -> To Workspace2/1, Scope/1, Sum/1  "VOC"
  Gain/1 -> Sum/2
  Sum/1 -> Cells in series/1
  Cells in series/1 -> V_battery/1
  Integrator1/1 -> Divide/1
  Divide/1 -> Sum1/2
  Constant1/1 -> Sum1/1
  Unit Delay/1 -> Square/1, Gain/1
  Square/1 -> Gain1/1
  Gain1/1 -> Integrator/1, To Workspace/1
  Integrator/1 -> To Workspace1/1
  Constant/1 -> Gain2/1
  Gain2/1 -> Divide/2
  I_battery/1 -> MATLAB Function/1(I_batt)
  MATLAB Function/1(I_batt_min) -> Scope1/1, Cells in Parallel/1

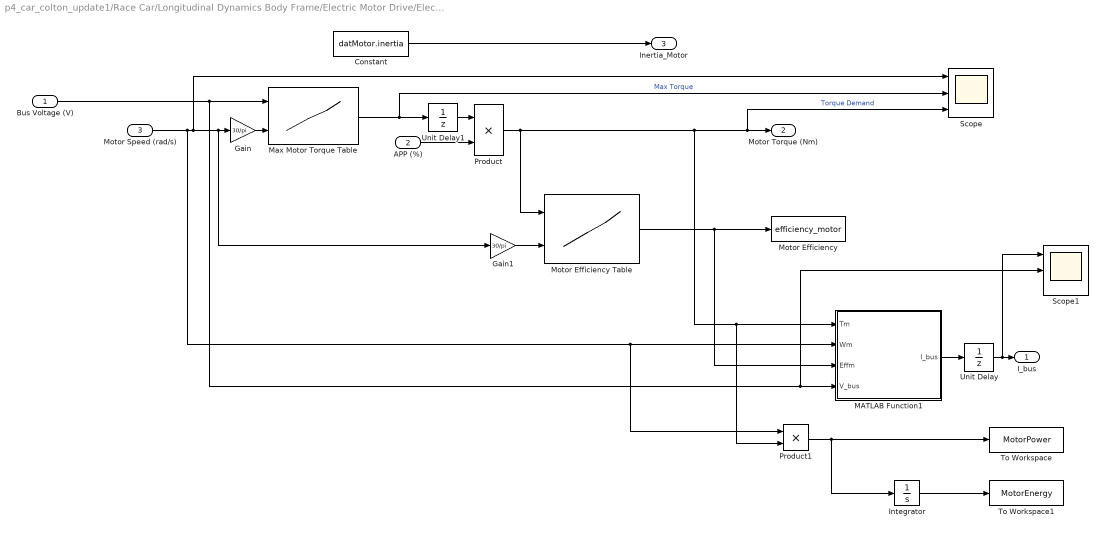
== system p4_car_colton_update1/Race Car/Longitudinal Dynamics Body Frame/Electric Motor Drive/Electric Motor ==
  Bus Voltage (V) : Inport
  APP (%) : Inport  Port=2
  Motor Speed (rad/s) : Inport  Port=3
  Constant : Constant  Value=datMotor.inertia
  Gain : Gain  Gain=30/pi
  Gain1 : Gain  Gain=30/pi
  Integrator : Integrator
  MATLAB Function1 : MATLAB Function  TreatAsAtomicUnit=on
  Max Motor Torque Table : Lookup_n-D  BreakpointsForDimension1=datMotor.vbus  BreakpointsForDimension2=datMotor.rpm  BreakpointsForDimension3=[5, 7]  Table=datMotor.maxtorque  ExtrapMethod=Clip  UseLastTableValue=on  InternalRulePriority=Speed  RndMeth=Simplest
      settings: InputPortMap=u0,u1
  Motor Efficiency : ToWorkspace  VariableName=efficiency_motor  SaveFormat=Timeseries  SampleTime=-1
  Motor Efficiency Table : Lookup_n-D  BreakpointsForDimension1=datMotor.eta_torque  BreakpointsForDimension2=datMotor.eta_speed  BreakpointsForDimension3=[5, 7]  Table=datMotor.eta_val  ExtrapMethod=Clip  UseLastTableValue=on  InternalRulePriority=Speed  RndMeth=Simplest
      settings: InputPortMap=u0,u1
  Product : Product
  Product1 : Product
  Scope : Scope  NumInputPorts=3
      settings: ActiveDisplayYMinimum=-117.53104  ActiveDisplayYMaximum=699.63306
  Scope1 : Scope  NumInputPorts=3
      settings: ActiveDisplayYMinimum=-70.21177  ActiveDisplayYMaximum=433.2973  DataLoggingVariableName=ScopeData2
  To Workspace : ToWorkspace  VariableName=MotorPower  SaveFormat=Timeseries  SampleTime=-1
  To Workspace1 : ToWorkspace  VariableName=MotorEnergy  SaveFormat=Timeseries  SampleTime=-1
  Unit Delay : UnitDelay  SampleTime=-1  HasFrameUpgradeWarning=on
  Unit Delay1 : UnitDelay  SampleTime=-1  HasFrameUpgradeWarning=on
  I_bus : Outport
  Motor Torque (Nm) : Outport  Port=2
  Inertia_Motor : Outport  Port=3
  wires:
  Max Motor Torque Table/1 -> Unit Delay1/1, Scope/2  "Max Torque"
  Constant/1 -> Inertia_Motor/1
  APP (%)/1 -> Product/2
  Product/1 -> Product1/2, MATLAB Function1/1(Tm), Scope/3, Motor Torque (Nm)/1, Motor Efficiency Table/1  "Torque Demand"
  Motor Efficiency Table/1 -> Motor Efficiency/1, MATLAB Function1/3(Effm)
  MATLAB Function1/1(I_bus) -> Unit Delay/1
  Unit Delay/1 -> Scope1/1, I_bus/1
  Product1/1 -> Integrator/1, To Workspace/1
  Integrator/1 -> To Workspace1/1
  Gain/1 -> Max Motor Torque Table/2
  Gain1/1 -> Motor Efficiency Table/2
  Motor Speed (rad/s)/1 -> Product1/1, MATLAB Function1/2(Wm), Scope/1, Gain1/1, Gain/1
  Bus Voltage (V)/1 -> Scope1/2, MATLAB Function1/4(V_bus), Max Motor Torque Table/1
  Unit Delay1/1 -> Product/1

== system p4_car_colton_update1/Race Car/Longitudinal Dynamics Body Frame/Electric Motor Drive/Inverter ==
  V_battery : Inport
  I_bus : Inport  Port=2
  Efficiency Inverter : Constant  Value=0.95
  Inverter Calculations : MATLAB Function  TreatAsAtomicUnit=on
  V_bus : Outport
  I_battery : Outport  Port=2
  wires:
  V_battery/1 -> Inverter Calculations/1(V_bat)
  Inverter Calculations/1(V_bus) -> V_bus/1
  Efficiency Inverter/1 -> Inverter Calculations/2(Eff_I)
  I_bus/1 -> Inverter Calculations/3(I_bus)
  Inverter Calculations/2(I_bat) -> I_battery/1

== system p4_car_colton_update1/Race Car/Longitudinal Dynamics Body Frame/Vehicle/vehicleDragForce ==
  vel : Inport
  Drag Force : MATLAB Function  TreatAsAtomicUnit=on
  To Workspace : ToWorkspace  VariableName=Faero  SaveFormat=Timeseries  SampleTime=-1
  drag coeff : Constant  Value=datCar.C2
  rolling friction coeff : Constant  Value=datCar.C1
  static friction : Constant  Value=datCar.C0
  Fdrag : Outport
  wires:
  static friction/1 -> Drag Force/1(C0)
  Drag Force/1(Fdrag) -> Fdrag/1, To Workspace/1
  vel/1 -> Drag Force/4(vel)
  rolling friction coeff/1 -> Drag Force/2(C1)
  drag coeff/1 -> Drag Force/3(C2)

== system p4_car_colton_update1/Race Car/Longitudinal Dynamics Body Frame/Vehicle/vehicleDynamics ==
  "Fw " : Inport
  Fd : Inport  Port=2
  "M_in " : Inport  Port=3
  vy : Inport  Port=4
  omega : Inport  Port=5
  grade Percent : Inport  Port=6
  Constant3 : Constant  Value=datCar.m
  Integrator : Integrator  InitialCondition=datCar.init.vx0  LimitOutput=on  LowerSaturationLimit=0
  MATLAB Function : MATLAB Function  TreatAsAtomicUnit=on
  Scope : Scope
      settings: ActiveDisplayYMinimum=-1  ActiveDisplayYMaximum=1  DataLoggingVariableName=ScopeData18
  acceleration : Outport
  Out2 : Outport  Port=2
  wires:
  MATLAB Function/1(acceleration) -> Scope/1, acceleration/1, Integrator/1
  "Fw "/1 -> MATLAB Function/2(Fw)
  vy/1 -> MATLAB Function/5(Vy)
  "M_in "/1 -> MATLAB Function/4(M_in)
  Constant3/1 -> MATLAB Function/1(M)
  omega/1 -> MATLAB Function/6(Omega)
  Fd/1 -> MATLAB Function/3(Fd)
  Integrator/1 -> Out2/1
  grade Percent/1 -> MATLAB Function/7(gradePercent)

== matlab function p4_car_colton_update1/Race Car/CarLateralDynamicsBodyFrame/LateralDynamics ==
  data: Fyf input; Fyr input size=1; vx input; omega input; ay output; obj parameter; omega_dot output
function [ay, omega_dot] = fcn(Fyf, Fyr, vx, omega, obj)

Fy = Fyf + Fyr;
ay = Fy / obj.m - omega * vx;
        
M  = Fyf * obj.lf - Fyr * obj.lr;        
omega_dot = M / obj.I;        

end

== matlab function p4_car_colton_update1/Race Car/Longitudinal Dynamics Body Frame/Vehicle/vehicleDragForce/Drag Force ==
  data: C0 input; Fdrag output; C1 input; C2 input; vel input
function Fdrag = drag(C0, C1, C2, vel)
    
Fdrag = C0 + C1*vel + C2*(vel)^2;

== matlab function p4_car_colton_update1/Race Car/Longitudinal Dynamics Body Frame/Vehicle/vehicleDynamics/MATLAB Function ==
  data: M input; Fw input; Fd input; acceleration output; M_in input; Vy input; Omega input; gradePercent input
function acceleration = vehicle(M, Fw, Fd, M_in, Vy, Omega, gradePercent)


g = 9.81; %m/s/s
acceleration = ((Fw - Fd - M * g * sin(atan(gradePercent))) ...
    / (M + M_in)) + Vy*Omega;

== matlab function p4_car_colton_update1/Race Car/CarLateralDynamicsBodyFrame/TireForces ==
  data: alpha_f input; alpha_r input; Fyf output; obj parameter; Fyr output
function [Fyf, Fyr] = fcn(alpha_f, alpha_r, obj)

Fyf = max(-obj.Fyfmax, min(obj.Fyfmax, obj.Calpha_f * alpha_f));
Fyr = max(-obj.Fyrmax, min(obj.Fyrmax, obj.Calpha_r * alpha_r));

end

== matlab function p4_car_colton_update1/Race Car Driver/Throttle and Braking Logic /MATLAB Function ==
  data: a input; APP output; b input; v input; BPP output; SOC input; regen output
function [APP, BPP, regen] = fcn(a, b, v, SOC)
% a = accel request in [0..1]  (max(PP,0))
% b = brake  request in [0..1]  (max(-PP,0))
% v = vehicle speed [m/s], SOC in [0..1]

    % Speed thresholds for regen (5 mph to 25 mph)
    mph2mps = 0.44704;
    speed1 = 5  * mph2mps;
    speed2 = 25 * mph2mps;
    dspeed = max(speed2 - speed1, 1e-6);

    % Base regen fraction vs speed
    absv = abs(v);
    if absv < speed1
        regen = 0;
    elseif absv <= speed2
        regen = 0.95 * (absv - speed1) / dspeed;
    else
        regen = 0.95;
    end

    % SOC derate: full regen ≤ 80%, taper to 0 at 100%
    if SOC <= 0.8
        SOCfactor = 1;
    elseif SOC < 1
        SOCfactor = 1 - (SOC - 0.8) / 0.2;
    else
        SOCfactor = 0;
    end

    regen = regen * SOCfactor;
    
    % Final pedal/commands
    APP = a;                      % accelerator is ONLY the positive request
    BPP = b * (1 - regen);        % friction brake handles what regen can't
    % 'regen' is the regen fraction of the brake request (0..0.95)
end

== matlab function p4_car_colton_update1/Race Car/Longitudinal Dynamics Body Frame/Electric Motor Drive/Battery/MATLAB Function ==
  data: I_batt input; SOC input; I_batt_min output
function I_batt_min = fcn(I_batt, SOC)
    if SOC <= 0.1
        I_batt_min = 0;
    else
        I_batt_min = I_batt;
    end

== matlab function p4_car_colton_update1/Race Car Driver/Throttle and Braking Logic /MATLAB Function1 ==
  data: regen input; viol output; v input
function viol = fcn(regen, v)
    if v < (5*(1600/3600))
        regen_vio = 0;
        if regen == regen_vio
            viol = 0;
        else
            viol = 1;
        end

    elseif v == (25*(1600/3600))
        regen_vio = 0.95;
        if regen == regen_vio
            viol = 0;
        else
            viol = 1;
        end

    elseif v > (25*(1600/3600))
        regen_vio = 0.95;
        if regen == regen_vio
            viol = 0;
        else
            viol = 1;
        end
    else
        regen_vio = (0.95/20)*v;
        if regen == regen_vio
            viol = 0;
        else
            viol = 1;
        end
    end

%     BRK = BPP * -1;
%     if(BRK >= 0) && (1 >= BRK)
%         viol = 0;
%     else
%         viol = 1;
%     end

== matlab function p4_car_colton_update1/Race Car/CarLateralDynamicsBodyFrame/TireSlip ==
  data: vy input size=1; vx input; delta_f input size=1; omega input; alpha_f output; obj parameter; alpha_r output
function [alpha_f, alpha_r] = fcn(vy,  vx, delta_f, omega, obj)


if abs(vx)> obj.vx_threshold1
      alpha_f = delta_f - (vy + omega * obj.lf) / vx;
      alpha_r = - (vy - omega * obj.lr) / vx;
else
      alpha_f = 0;
      alpha_r = 0;
end



end

== matlab function p4_car_colton_update1/Race Car/Longitudinal Dynamics Body Frame/Drive/Transmission ==
  data: t_trans_in input; I_trans_in input; gear_ratio input; I_trans input; t_trans_out output; I_trans_out output; omega_trans_out input; alpha_trans_out input; omega_trans_in output; alpha_trans_in output
function [t_trans_out,  I_trans_out, omega_trans_in, alpha_trans_in]= ...
        transmission(t_trans_in, I_trans_in,  ...
        gear_ratio, I_trans, omega_trans_out, alpha_trans_out)

t_trans_out = t_trans_in * gear_ratio ;
I_trans_out = (I_trans_in + I_trans)* gear_ratio^2;
omega_trans_in = omega_trans_out * gear_ratio;
alpha_trans_in = alpha_trans_out * gear_ratio;

end

== matlab function p4_car_colton_update1/Race Car Driver/Driver/MATLAB Function ==
  data: x input; delta output; y input; yaw input; xpath input; ypath input; Vxd1 output; tpath input; lookahead input; lf input; lr input
function [delta, Vxd1] = driver(x, y, yaw, xpath, ypath, tpath, lookahead, lf, lr)
% DRIVER computes steering angle (delta) and desired speed (Vxd1)
% Continuous-time, no persistent state.
% Uses heading change within the lookahead arc; ignores 'radius'.

% =========================
% Parameters
% =========================
Vmax = 45 * 0.44704;   % [m/s] 45 mph
Vmin = 10 * 0.44704;   % [m/s] 10 mph
L    = lf + lr;        % wheelbase [m]

% =========================
% 1) Nearest path point
% =========================
dist2    = (xpath - x).^2 + (ypath - y).^2;
[~, idx] = min(dist2);
N        = numel(xpath);
if N < 2
    delta = 0; Vxd1 = Vmin; return;
end

% =========================
% 2) Arc-length coordinate + lookahead target
% =========================
s_path  = [0; cumsum(hypot(diff(xpath), diff(ypath)))];
L_total = s_path(end);

s_now  = s_path(idx);
s_goal = s_now + lookahead;
if s_goal > L_total
    s_goal = s_goal - L_total;  % wrap around
end

% Interpolate target point on path
x_target = interp1(s_path, xpath, s_goal, 'linear', 'extrap');
y_target = interp1(s_path, ypath, s_goal, 'linear', 'extrap');

% =========================
% 3) Pure-pursuit steering
% =========================
dx   = x_target - x;
dy   = y_target - y;
Ld   = max(hypot(dx, dy), 1e-6);          % geometric distance to target
alpha = atan2(dy, dx) - yaw;              % heading error to target
alpha = atan2(sin(alpha), cos(alpha));    % wrap to [-pi,pi]
delta_pp = atan2(2 * L * sin(alpha), Ld);

% =========================
% 4) Lateral error feedback (tighten line tracking)
% =========================
ex    = xpath(idx) - x;
ey    = ypath(idx) - y;
e_lat =  cos(yaw)*ey - sin(yaw)*ex;       % signed cross-track error
k_lat = 0.8;                              % stronger than before
delta_lat = atan(k_lat * e_lat / max(Ld, 1));

% =========================
theta_unwrap = unwrap(tpath(:));                                
theta_now    = theta_unwrap(max(1, min(idx, numel(theta_unwrap))));
theta_goal   = interp1(s_path, theta_unwrap, s_goal, 'linear', 'extrap');

% Signed heading change in [-pi,pi]
dtheta   = atan2( sin(theta_goal - theta_now), cos(theta_goal - theta_now) );
% Preview curvature κ ≈ Δθ / Δs  (Δs ≈ lookahead by construction)
kappa_ff = dtheta / max(lookahead, 1e-6);                       % [1/m]
delta_ff = L * kappa_ff;                                        % steering 

% =========================
% 6) Combine & smooth-limit 
% =========================
lookahead_gain = 10 / (lookahead + 1);   % smaller lookahead ⇒ stronger response
delta_raw = (1 + 0.25*lookahead_gain) * (delta_pp + 0.5*delta_lat) + 1.0*delta_ff;
delta     = 0.7 * tanh(delta_raw / 0.7); % smooth saturation (±~0.7 rad)

% =========================
% Turn intensity from the same dtheta preview
theta_ref    = pi/6;                                            % ≈30° over lookahead
curve_factor = min(1.0, max(0.0, abs(dtheta) / theta_ref));     % 0..1
Vxd1         = Vmax - (Vmax - Vmin) * curve_factor;             % map to [Vmin,Vmax]

end

== matlab function p4_car_colton_update1/Race Car/Longitudinal Dynamics Body Frame/Drive/Final Drive ==
  data: t_trans_in input; I_trans_in input; gear_ratio input; I_trans input; t_trans_out output; I_trans_out output; omega_trans_out input; alpha_trans_out input; omega_trans_in output; alpha_trans_in output
function [t_trans_out, I_trans_out, omega_trans_in, alpha_trans_in]= ...
        finalDrive(t_trans_in, I_trans_in,  ...
        gear_ratio, I_trans, omega_trans_out, alpha_trans_out)

t_trans_out = t_trans_in * gear_ratio ;
I_trans_out = (I_trans_in + I_trans)* gear_ratio^2;
omega_trans_in = omega_trans_out * gear_ratio;
alpha_trans_in = alpha_trans_out * gear_ratio;

end

== matlab function p4_car_colton_update1/Environment/MATLAB Function ==
  data: x input; g output; y input
function g = trackGrade(x, y)
% Returns the local grade at position (x,y) along the track.
% Positive values indicate uphill, negative values downhill.

    % Intermediate variable for slope shaping along the straight
    u = (x - 450) / 50;

    % Derivative of the elevation function (supplied in project spec)
    Slope = 0.2 * exp(u) ./ (1 + exp(u)).^2;

    % --- Determine grade based on track section ---
    if y < 200
        % Lower straight section
        if x <= 0 || x >= 900
            g = 0;       % both curves are level
        else
            g = Slope;   % rising grade
        end

    elseif y > 200
        % Upper straight section
        if x <= 0 || x >= 900
            g = 0;        % curves remain flat
        else
            g = -Slope;   % descending grade
        end

    else
        % In case of boundary overlap, treat as zero grade
        g = 0;
    end
end

== matlab function p4_car_colton_update1/Race Car/Longitudinal Dynamics Body Frame/Electric Motor Drive/Electric Motor/MATLAB Function1 ==
  data: Tm input; I_bus output; Wm input; Effm input; V_bus input
function I_bus = fcn(Tm, Wm, Effm, V_bus)
    Pm = Tm*Wm;
    sgn_m = Pm / (abs(Pm) + 0.001);
    Pe = Pm / (Effm^sgn_m);
    if V_bus > 1
        I_bus = Pe/V_bus;
    else
        I_bus = 0;
    end

== matlab function p4_car_colton_update1/Race Car/Longitudinal Dynamics Body Frame/Wheel /MATLAB Function ==
  data: r_w input; v_w input; omega_w input; lambda output
function lambda = tire_slip_ratio(r_w, v_w, omega_w)
% r_w - wheel radius
% v_w - wheel axle speed (m/s)
% omega_w - wheel speed (rad/s)
% lambda - tire slip ratio

epsilon = 0.0001; % a small number for numerical smoothening

if (r_w * omega_w >= v_w - epsilon)
    lambda = (r_w * omega_w - v_w) / (abs(r_w * omega_w) + epsilon);
else
    lambda = (r_w * omega_w - v_w) / (abs(v_w) + epsilon);
end

== matlab function p4_car_colton_update1/Race Car/Longitudinal Dynamics Body Frame/Wheel /MATLAB Function1 ==
  data: tau_axle input; alpha_w output; tau_brake input; I_in input; I_w input; r_w input; F_x input
function alpha_w = wheel_acceleration(tau_axle, tau_brake, I_in, I_w, r_w, F_x)
% tau_axle - axle torque (Nm)
% tau_brake - brake torque (Nm)
% I_in - input inertia (Kg m^2)
% I_w - wheel inertia (Kg m^2)
% r_w - tire radius (m)
% F_x - tractive force from tire contact (N)
% alpha_w = wheel (angular) acceleration (rad / s^2)

alpha_w = (tau_axle - tau_brake - F_x * r_w ) / (I_in + I_w);

== matlab function p4_car_colton_update1/Race Car/Longitudinal Dynamics Body Frame/Wheel /MATLAB Function2 ==
  data: lambda input; F_x output; lambda_max input; nominal_stiffness input; mu input; mass input
function F_x = tire_tractive_force(lambda, lambda_max, nominal_stiffness, mu, mass )
% lambda - tire slip ratio
% lambda_max - maximum tire slip ratio for F_x calculations
% nominal_stiffness - tire long stiffness (N)
% mu - (effective) friction coefficient - in the range [0, 1]
% mass - vehicle mass for normal force calculation

g = 9.81; % gravity - m/ s^2

N = mass * g/4;  % assume 4 tires and equal distribution across tires

C_lambda = nominal_stiffness * mu * N;
if lambda >= 0
    F_x = C_lambda * min(lambda_max, lambda);
else
    F_x = C_lambda * max(-lambda_max, lambda);
end

== matlab function p4_car_colton_update1/Race Car/Longitudinal Dynamics Body Frame/Electric Motor Drive/Inverter/Inverter Calculations ==
  data: V_bat input; Eff_I input; V_bus output; I_bus input; I_bat output
function [V_bus, I_bat] = fcn(V_bat, Eff_I, I_bus)
    V_bus = V_bat; % Vbus = Vbat * r, where r is the inverter conversion ratio % * I_bat * Eff_I^(sgn_Pbat))/ I_bus;
    P_bus = V_bus *I_bus;
    sgn_Pbus = P_bus / (abs(P_bus) + 0.001);
    
    if V_bat > 1
        I_bat = (P_bus / Eff_I^sgn_Pbus) / V_bat ;
    else
        I_bat = 0;
    end

end

% double check

== matlab function p4_car_colton_update1/Race Car/CarKinematicsInertialFrame/KinematicVehicleModel_derivatives ==
  data: vx input; vy input; psi input size=1; Xdot output; Ydot output
function [Xdot, Ydot] = fcn(vx, vy, psi)
    temp = TF(psi) * [vx;vy]; 
    Xdot = temp(1);
    Ydot = temp(2);
  
end

function y = TF(psi)
    y = [cos(psi), -sin(psi); sin(psi), cos(psi)];
end

== matlab function p4_car_colton_update1/Race Car/Longitudinal Dynamics Body Frame/Brake System/Brake Torque ==
  data: BBcmd input; Tbcap input; Tb output; w_wheel input
function Tb = fcn(BBcmd, Tbcap, w_wheel)
% DESCRIPTION: 
%   This function takes the brake torque capacity, the angular velocity of
%   the wheel. A simple approximation for the brake torque capacity is 
%   the brake command times some calibratable constant 

% INPUTS:
%   BBcmd - brake percent command
%   Tbcap - brake torque capacity  [N-m]
%   w_wheel - wheels angular velocity [rad/s]

% OUTPUTS:
%   Tb - actual brake torque [N-m]

Tb = -BBcmd * Tbcap * (w_wheel / (abs(w_wheel) + 0.001));

end
